simulink model "psbtwelvepulses"  (Simulink 6.0)
settings: Solver=ode23tb  StartTime=0.0  StopTime=.05  RelTol=1e-3
InitFcn:
  | powericon('psbinitsys',bdroot);
undefined symbols (not defined in the file or in its folder): D1, Delta
libraries: powerlib2 x18, powerlib_extras x1
settings Model: Creator=dkennedy  LastModifiedBy=batserve  ExtModeAutoUpdateStatusClock=off
settings DataIOCC: SignalLoggingName=sigsOut
settings OptimizationCC: BlockReduction=off  BooleanDataType=off
settings DebuggingCC: SolverPrmCheckMsg=none
settings HardwareCC: TargetUnknown=on

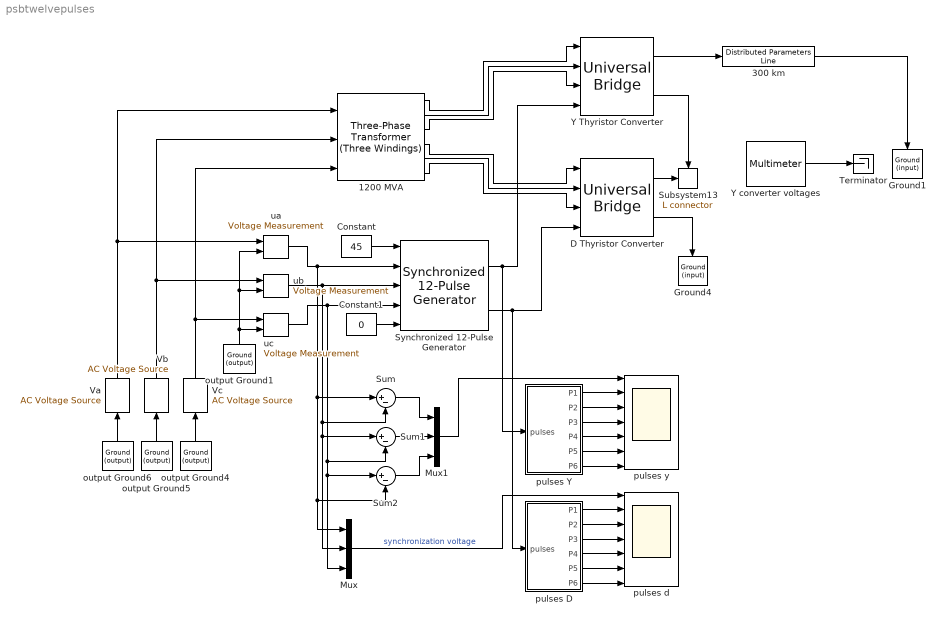
== system psbtwelvepulses ==
  " Synchronized 12-Pulse Generator" : powerlib_extras/Control  Blocks/ Synchronized 12-Pulse Generator  freq=60  pwidth=20  Double_Pulse=off
  1200 MVA : powerlib2/Elements/Three-Phase Transformer (Three Windings)  Tag=PoWeRsYsTeMbLoCk  confi=ABC as input terminals  nom=[ 1200e6 , 60 ]  ydw1=Yg  w1="[ 500e3 0  0 ]"  ydw2=Y  w2=[ 200e3 0 0]  ydw3=Delta (D1)  w3=[ 200e3 0.001 0]  ynsat=off  rmag=500  lm=500  sat=[0 0; 1 1.2; 2 1.1]  hyst=off  matfile='basic_model'  sif=off  ifl=[0.8 -0.8 0.7]  initialslopes=[+1 +1 +1]  mesure=None  PSBOutputType=111111
  300 km : powerlib2/Elements/Distributed Parameters Line  Tag=PoWeRsYsTeMbLoCk  n=1  f=60  r=0.015  l=0.792e-3  c=14.4e-9  lgt=300  x1=[0 0 0 0; 0.0001244 0 0 0; 0.0002488 0 0 0; 0.0003733 0 0 0; 0.0004977 0 0 0; 0.0006221 0 0 0]  x2=[0 0 0 0; 0.0001244 0 0 0; 0.0002488 0 0 0; 0.0003733 0 0 0; 0.0004977 0 0 0; 0.0006221 0 0 0]  x3=[0 0 0 0; 0.0001244 0 0 0; 0.0002488 0 0 0; 0.0003733 0 0 0; 0.0004977 0 0 0; 0.0006221 0 0 0]  x4=[0 0 0 0; 0.0001244 0 0 0; 0.0002488 0 0 0; 0.0003733 0 0 0; 0.0004977 0 0 0; 0.0006221 0 0 0]  x5=0  mesure=Phase-to-ground voltages  PSBOutputType=111111111111111111111111111111
  Constant : Constant  Value=45
  Constant1 : Constant  Value=0
  D Thyristor Converter : powerlib2/Power Electronics/Universal Bridge  Tag=PoWeRsYsTeMbLoCk  arms=3  confi=ABC as input terminals  injcc=2000  cf=inf  device=Thyristors  Ron=1e-3  Lon=0  VFs="[  0.8  0.8  ]"  Vf=0  gtoparameters=[ 10e-6 , 20e-6 ]  igbtparameters=[ 1e-6 , 2e-6 ]  mesure=All voltages and currents  PSBOutputType=111
  Ground1 : powerlib2/Connectors/Ground (input)  Tag=PoWeRsYsTeMbLoCk  Orientation=down
  Ground4 : powerlib2/Connectors/Ground (input)  Tag=PoWeRsYsTeMbLoCk  Orientation=down
  Mux : Mux  Inputs=3
  Mux1 : Mux  Inputs=3
  Subsystem13 : powerlib2/Connectors/L connector  Tag=PoWeRsYsTeMbLoCk
  Sum : Sum  Inputs=|+-  SaturateOnIntegerOverflow=on  InputSameDT=on
  Sum1 : Sum  Inputs=|+-  SaturateOnIntegerOverflow=on  InputSameDT=on
  Sum2 : Sum  Inputs=|+-  SaturateOnIntegerOverflow=on  InputSameDT=on
  Terminator : Terminator
  Va : powerlib2/Electrical Sources/AC Voltage Source  Tag=PoWeRsYsTeMbLoCk  Orientation=up  A=500e3/sqrt(3)*sqrt(2)  P=0  F=60  stime=0  mesure=None  PSBOutputType=1
  Vb : powerlib2/Electrical Sources/AC Voltage Source  Tag=PoWeRsYsTeMbLoCk  Orientation=up  A=500e3/sqrt(3)*sqrt(2)  P=-120  F=60  stime=0  mesure=None  PSBOutputType=1
  Vc : powerlib2/Electrical Sources/AC Voltage Source  Tag=PoWeRsYsTeMbLoCk  Orientation=up  A=500e3/sqrt(3)*sqrt(2)  P=120  F=60  stime=0  mesure=None  PSBOutputType=1
  Y Thyristor Converter : powerlib2/Power Electronics/Universal Bridge  Tag=PoWeRsYsTeMbLoCk  arms=3  confi=ABC as input terminals  injcc=2000  cf=.1e-6  device=Thyristors  Ron=1e-3  Lon=0  VFs="[  0.8  0.8  ]"  Vf=0  gtoparameters=[ 10e-6 , 20e-6 ]  igbtparameters=[ 1e-6 , 2e-6 ]  mesure=All voltages and currents  PSBOutputType=111
  "Y converter voltages " : powerlib2/Measurements/Multimeter  Tag=PoWeRsYsTeMmEaSuReMeNt  PhasorSimulation=off  OutputType=Magnitude  sel=[1 2 3 4 5 6 19]  L=32  Gain=[-1 -1 -1 -1 -1 -1 1]  yselected={'Usw1: D Thyristor Converter','Usw2: D Thyristor Converter','Usw3: D Thyristor Converter','Usw4: D Thyristor Converter','Usw5: D Thyristor Converter','Usw6: D Thyristor Converter','Us_ph1_gnd: 300 km'};  PSBOutputType=1  PSBequivalent=0  AxesSetting=[0,0.1,-100,100]  Display=1  SavedBlockNames=-11
  output Ground{1,4..6} (4 alike) : powerlib2/Connectors/Ground (output)  Tag=PoWeRsYsTeMbLoCk  Orientation=up  PSBOutputType=1
  pulses D : Subsystem
  pulses Y : Subsystem
  pulses d : Scope  NumInputPorts=7
      settings: TimeRange=0.035  YMin=-500000~0~0~0~0~0~0  YMax=500000~1~1~1~1~1~1  SaveName=VI_scope1  SampleInput=on  SampleTime=1/60/512
  pulses y : Scope  NumInputPorts=7
      settings: TimeRange=0.1  YMin=-500000~0~0~0~0~0~0  YMax=500000~1~1~1~1~1~1  SaveName=VI_scope  SampleInput=on  SampleTime=1/60/512
  ua : powerlib2/Measurements/Voltage Measurement  Tag=PoWeRsYsTeMmEaSuReMeNt  PhasorSimulation=off  OutputType=Magnitude  PSBOutputType=0  PSBequivalent=0
  ub : powerlib2/Measurements/Voltage Measurement  Tag=PoWeRsYsTeMmEaSuReMeNt  PhasorSimulation=off  OutputType=Magnitude  PSBOutputType=0  PSBequivalent=0
  uc : powerlib2/Measurements/Voltage Measurement  Tag=PoWeRsYsTeMmEaSuReMeNt  PhasorSimulation=off  OutputType=Magnitude  PSBOutputType=0  PSBequivalent=0
  wires:
  output Ground6/1 -> Va/1
  output Ground5/1 -> Vb/1
  output Ground4/1 -> Vc/1
  Vc/1 -> uc/1, 1200 MVA/3
  Vb/1 -> ub/1, 1200 MVA/2
  Va/1 -> ua/1, 1200 MVA/1
  output Ground1/1 -> ua/2, ub/2, uc/2
  ua/1 -> " Synchronized 12-Pulse Generator"/2, Sum/1, Mux/1, Sum2/2
  ub/1 -> " Synchronized 12-Pulse Generator"/3, Sum/2, Mux/2, Sum1/1
  uc/1 -> " Synchronized 12-Pulse Generator"/4, Sum1/2, Mux/3, Sum2/1
  Constant1/1 -> " Synchronized 12-Pulse Generator"/5
  D Thyristor Converter/1 -> Subsystem13/1
  D Thyristor Converter/2 -> Ground4/1
  1200 MVA/2 -> Y Thyristor Converter/2
  1200 MVA/1 -> Y Thyristor Converter/1
  1200 MVA/3 -> Y Thyristor Converter/3
  " Synchronized 12-Pulse Generator"/1 -> Y Thyristor Converter/4, pulses Y/1(pulses)
  " Synchronized 12-Pulse Generator"/2 -> D Thyristor Converter/4, pulses D/1(pulses)
  Y Thyristor Converter/2 -> Subsystem13/Enable
  Y Thyristor Converter/1 -> 300 km/1
  300 km/1 -> Ground1/1
  pulses D/6(P6) -> pulses d/7
  pulses D/1(P1) -> pulses d/2
  pulses D/2(P2) -> pulses d/3
  pulses D/3(P3) -> pulses d/4
  pulses D/4(P4) -> pulses d/5
  pulses D/5(P5) -> pulses d/6
  Mux/1 -> pulses d/1  "synchronization voltage"
  Sum/1 -> Mux1/1
  Sum1/1 -> Mux1/2
  Sum2/1 -> Mux1/3
  Mux1/1 -> pulses y/1
  "Y converter voltages "/1 -> Terminator/1
  Constant/1 -> " Synchronized 12-Pulse Generator"/1
  pulses Y/1(P1) -> pulses y/2
  pulses Y/2(P2) -> pulses y/3
  pulses Y/3(P3) -> pulses y/4
  pulses Y/4(P4) -> pulses y/5
  pulses Y/5(P5) -> pulses y/6
  pulses Y/6(P6) -> pulses y/7
  1200 MVA/4 -> D Thyristor Converter/1
  1200 MVA/5 -> D Thyristor Converter/2
  1200 MVA/6 -> D Thyristor Converter/3

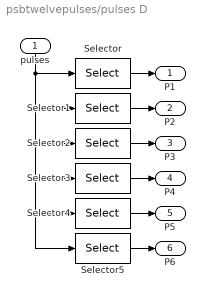
== system psbtwelvepulses/pulses D ==
  pulses : Inport  Orientation=down  Port=1  LatchInput=off
  Selector : Selector  InputPortWidth=6
  Selector1 : Selector  Elements=2  InputPortWidth=6
  Selector2 : Selector  Elements=3  InputPortWidth=6
  Selector3 : Selector  Elements=4  InputPortWidth=6
  Selector4 : Selector  Elements=5  InputPortWidth=6
  Selector5 : Selector  Elements=6  InputPortWidth=6
  P1 : Outport
  P2 : Outport  Port=2
  P3 : Outport  Port=3
  P4 : Outport  Port=4
  P5 : Outport  Port=5
  P6 : Outport  Port=6
  wires:
  Selector/1 -> P1/1
  pulses/1 -> Selector4/1, Selector5/1, Selector3/1, Selector2/1, Selector1/1, Selector/1
  Selector1/1 -> P2/1
  Selector2/1 -> P3/1
  Selector3/1 -> P4/1
  Selector4/1 -> P5/1
  Selector5/1 -> P6/1

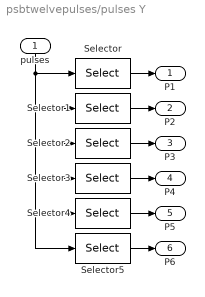
== system psbtwelvepulses/pulses Y ==
  pulses : Inport  Orientation=down  Port=1  LatchInput=off
  Selector : Selector  InputPortWidth=6
  Selector1 : Selector  Elements=2  InputPortWidth=6
  Selector2 : Selector  Elements=3  InputPortWidth=6
  Selector3 : Selector  Elements=4  InputPortWidth=6
  Selector4 : Selector  Elements=5  InputPortWidth=6
  Selector5 : Selector  Elements=6  InputPortWidth=6
  P1 : Outport
  P2 : Outport  Port=2
  P3 : Outport  Port=3
  P4 : Outport  Port=4
  P5 : Outport  Port=5
  P6 : Outport  Port=6
  wires:
  Selector5/1 -> P6/1
  Selector4/1 -> P5/1
  Selector3/1 -> P4/1
  Selector2/1 -> P3/1
  Selector1/1 -> P2/1
  pulses/1 -> Selector/1, Selector1/1, Selector2/1, Selector3/1, Selector5/1, Selector4/1
  Selector/1 -> P1/1
